simulink model "generic_IVS"  (R2024a)
settings: Solver=FixedStepDiscrete  StartTime=0.0  StopTime=inf  FixedStep=0.001  RelTol=1e-3  EnableMultiTasking=on
undefined symbols (not defined in the file): filtered_route_waypoint_raw, route1_waypoint_x, route1_waypoint_y, route2_waypoint_raw, route2_waypoint_x, route2_waypoint_y, route3_waypoint_x, route3_waypoint_y, route4_waypoint_x, route4_waypoint_y, route5_waypoint_x, route5_waypoint_y
libraries: CarMaker4SL x125, slpidlib x7, simulink x1, robotalgslib x1
(part 3 of 5)

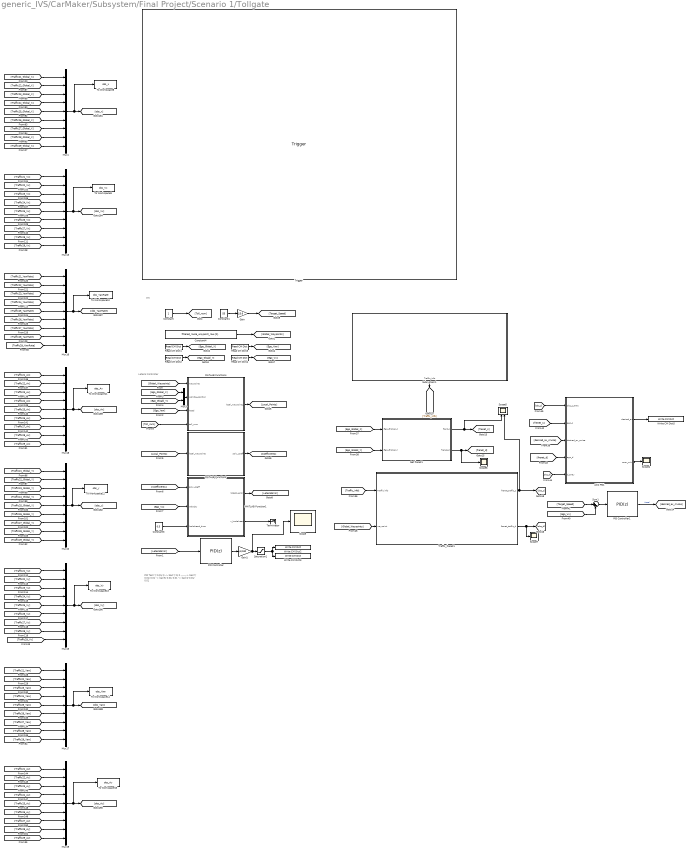
== system generic_IVS/CarMaker/Subsystem/Final Project/Scenario 1/Tollgate ==
  note: Lateral Controller
  note: Init
  note: PID Test
      | 7/ 0.01/ 0 -> bad
      | 7/ 0/ 0 ------> bad
      | 7/ 0.01/ 0.01 -> bad
      | 5/ 0.01/ 0.01 -> bad
      | 3/ 0.01/ 0.01
  Trigger : TriggerPort  TriggerType=function-call  VariantControl=(inherit)  PortDimensions=1
  ACC PD1 : MATLAB Function  TreatAsAtomicUnit=on
  Constant : Constant
  Constant1 : Constant  Value=55
  Constant3 : Constant  Value=0.5
  Constant4 : Constant  Value=filtered_route_waypoint_raw{2}
  Gain : Gain  Gain=1/3.6
  Gain1 : Gain  Gain=pi/180
  Get frenet1 : Subsystem
  MATLAB Function1 : MATLAB Function  TreatAsAtomicUnit=on
  MATLAB Function3 : MATLAB Function  TreatAsAtomicUnit=on
  "MATLAB Function4 " : MATLAB Function  TreatAsAtomicUnit=on
  Mux{1,10,13,15..19} (8 alike) : Mux  Inputs=9
  Mux3 : Mux  Inputs=2
  PID Controller : slpidlib/PID Controller  Controller=PID  Form=Parallel  TimeDomain=Discrete-time  UseExternalTs=off  SampleTime=-1  IntegratorMethod=Forward Euler  FilterMethod=Forward Euler  ControllerParametersSource=internal  P=3  I=0  UseKiTs=off  D=0.01  UseExternalDerivativeSource=off  N=3  UseFilter=on  TunerSelectOption=Transfer Function Based (PID Tuner App)  ZeroCross=off  InitialConditionSource=internal  InitialConditionForIntegrator=0  InitialConditionForFilter=0  DifferentiatorICPrevScaledInput=0  ExternalReset=none  TrackingMode=off  Kt=1  LimitOutput=off  SatLimitsSource=internal  UpperSaturationLimit=inf  LowerSaturationLimit=-inf  LinearizeAsGain=on  AntiWindupMode=none  Kb=1  LimitIntegrator=off  UpperIntegratorSaturationLimit=inf  LowerIntegratorSaturationLimit=-inf  POutMin=[]  POutMax=[]  IOutMin=[]  IOutMax=[]  DOutMin=[]  DOutMax=[]  NOutMin=[]  NOutMax=[]  SumOutMin=[]  SumOutMax=[]  SaturationOutMin=[]  SaturationOutMax=[]  PParamMin=[]  PParamMax=[]  IParamMin=[]  IParamMax=[]  DParamMin=[]  DParamMax=[]  NParamMin=[]  NParamMax=[]  KbParamMin=[]  KbParamMax=[]  KtParamMin=[]  KtParamMax=[]  KbOutMin=[]  KbOutMax=[]  KtOutMin=[]  KtOutMax=[]  IntegratorOutMin=[]  IntegratorOutMax=[]  FilterOutMin=[]  FilterOutMax=[]  SumI1OutMin=[]  SumI1OutMax=[]  SumI2OutMin=[]  SumI2OutMax=[]  SumI3OutMin=[]  SumI3OutMax=[]  SumI4OutMin=[]  SumI4OutMax=[]  SumDOutMin=[]  SumDOutMax=[]  DifferentiatorOutMin=[]  DifferentiatorOutMax=[]  FilterDiffOutCoefMin=[]  FilterDiffOutCoefMax=[]  ReciprocalOutMin=[]  ReciprocalOutMax=[]  SumDenOutMin=[]  SumDenOutMax=[]  SumNumOutMin=[]  SumNumOutMax=[]  DivideOutMin=[]  DivideOutMax=[]  UdiffTsProdOutMin=[]  UdiffTsProdOutMax=[]  NTsProdOutMin=[]  NTsProdOutMax=[]  UintegralTsProdOutMin=[]  UintegralTsProdOutMax=[]  UngainTsProdOutMin=[]  UngainTsProdOutMax=[]  ClampingZeroOutDataTypeStr=Inherit: Inherit via back propagation  ClampingZeroOutMin=[]  ClampingZeroOutMax=[]  FilterDenConstantOutDataTypeStr=Inherit: Inherit via back propagation  FilterDenConstantOutMin=[]  FilterDenConstantOutMax=[]  PCopyOutDataTypeStr=Inherit: Inherit via back propagation  PCopyOutMin=[]  PCopyOutMax=[]  NCopyOutDataTypeStr=Inherit: Inherit via back propagation  NCopyOutMin=[]  NCopyOutMax=[]  IntegratorContinuousStateAttributes=''  IntegratorStateMustResolveToSignalObject=off  IntegratorRTWStateStorageClass=Auto  FilterContinuousStateAttributes=''  FilterStateMustResolveToSignalObject=off  FilterRTWStateStorageClass=Auto  ParallelPVariant=InternalParameters  IdealPVariant=Disabled  IVariant=InternalParameters  DVariant=InternalParameters  IntegratorVariant=Discrete  SatVariant=Disabled  AWVariant=Passthrough  PCopyVariant=Disabled  TRVariant=Disabled  FdbkBlocksVariant=Forward  IdealPFdbkVariant=Disabled  SatFdbkVariant=Disabled  DerivativeFilterVariant=ForwardEulerFilter  NVariant=InternalParameters  NCopyVariant=Disabled  FilterICVariant=InternalICsFilter  IntegratorICVariant=InternalICs  ExternalResetVariant=Disabled  TRSumVariant=Passthrough  SumFdbkVariant=Disabled  SumVariant=Sum_PID  TsampFilterVariant=InternalTs  TsampNgainVariant=Passthrough  TsampIntegralVariant=Disabled_SignalSpec  ExternalSaturationOutDataTypeStr=Inherit: Same as second input  DerivativeSourceVariant=ErrorSignal
  PID Controller1 : slpidlib/PID Controller  Controller=PID  Form=Parallel  TimeDomain=Discrete-time  UseExternalTs=off  SampleTime=-1  IntegratorMethod=Forward Euler  FilterMethod=Forward Euler  ControllerParametersSource=internal  P=1  I=0  UseKiTs=off  D=0  UseExternalDerivativeSource=off  N=20  UseFilter=on  TunerSelectOption=Transfer Function Based (PID Tuner App)  InitialConditionSource=internal  InitialConditionForIntegrator=0  InitialConditionForFilter=0  DifferentiatorICPrevScaledInput=0  ExternalReset=none  TrackingMode=off  Kt=1  LimitOutput=off  SatLimitsSource=internal  UpperSaturationLimit=inf  LowerSaturationLimit=-inf  LinearizeAsGain=on  AntiWindupMode=none  Kb=1  LimitIntegrator=off  UpperIntegratorSaturationLimit=inf  LowerIntegratorSaturationLimit=-inf  POutMin=[]  POutMax=[]  IOutMin=[]  IOutMax=[]  DOutMin=[]  DOutMax=[]  NOutMin=[]  NOutMax=[]  SumOutMin=[]  SumOutMax=[]  SaturationOutMin=[]  SaturationOutMax=[]  PParamMin=[]  PParamMax=[]  IParamMin=[]  IParamMax=[]  DParamMin=[]  DParamMax=[]  NParamMin=[]  NParamMax=[]  KbParamMin=[]  KbParamMax=[]  KtParamMin=[]  KtParamMax=[]  KbOutMin=[]  KbOutMax=[]  KtOutMin=[]  KtOutMax=[]  IntegratorOutMin=[]  IntegratorOutMax=[]  FilterOutMin=[]  FilterOutMax=[]  SumI1OutMin=[]  SumI1OutMax=[]  SumI2OutMin=[]  SumI2OutMax=[]  SumI3OutMin=[]  SumI3OutMax=[]  SumI4OutMin=[]  SumI4OutMax=[]  SumDOutMin=[]  SumDOutMax=[]  DifferentiatorOutMin=[]  DifferentiatorOutMax=[]  FilterDiffOutCoefMin=[]  FilterDiffOutCoefMax=[]  ReciprocalOutMin=[]  ReciprocalOutMax=[]  SumDenOutMin=[]  SumDenOutMax=[]  SumNumOutMin=[]  SumNumOutMax=[]  DivideOutMin=[]  DivideOutMax=[]  UdiffTsProdOutMin=[]  UdiffTsProdOutMax=[]  NTsProdOutMin=[]  NTsProdOutMax=[]  UintegralTsProdOutMin=[]  UintegralTsProdOutMax=[]  UngainTsProdOutMin=[]  UngainTsProdOutMax=[]  ClampingZeroOutDataTypeStr=Inherit: Inherit via back propagation  ClampingZeroOutMin=[]  ClampingZeroOutMax=[]  FilterDenConstantOutDataTypeStr=Inherit: Inherit via back propagation  FilterDenConstantOutMin=[]  FilterDenConstantOutMax=[]  PCopyOutDataTypeStr=Inherit: Inherit via back propagation  PCopyOutMin=[]  PCopyOutMax=[]  NCopyOutDataTypeStr=Inherit: Inherit via back propagation  NCopyOutMin=[]  NCopyOutMax=[]  IntegratorContinuousStateAttributes=''  IntegratorStateMustResolveToSignalObject=off  IntegratorRTWStateStorageClass=Auto  FilterContinuousStateAttributes=''  FilterStateMustResolveToSignalObject=off  FilterRTWStateStorageClass=Auto  ParallelPVariant=InternalParameters  IdealPVariant=Disabled  IVariant=InternalParameters  DVariant=InternalParameters  IntegratorVariant=Discrete  SatVariant=Disabled  AWVariant=Passthrough  PCopyVariant=Disabled  TRVariant=Disabled  FdbkBlocksVariant=Forward  IdealPFdbkVariant=Disabled  SatFdbkVariant=Disabled  DerivativeFilterVariant=ForwardEulerFilter  NVariant=InternalParameters  NCopyVariant=Disabled  FilterICVariant=InternalICsFilter  IntegratorICVariant=InternalICs  ExternalResetVariant=Disabled  TRSumVariant=Passthrough  SumFdbkVariant=Disabled  SumVariant=Sum_PID  TsampFilterVariant=InternalTs  TsampNgainVariant=Passthrough  TsampIntegralVariant=Disabled_SignalSpec  ExternalSaturationOutDataTypeStr=Inherit: Same as second input  DerivativeSourceVariant=ErrorSignal
  Read CM Dict1 : CarMaker4SL/Read CM Dict  xname=Car.Fr1.tx  xsync=off  xstime=Inherited
  Read CM Dict2 : CarMaker4SL/Read CM Dict  xname=Car.Fr1.ty  xsync=off  xstime=Inherited
  Read CM Dict3 : CarMaker4SL/Read CM Dict  xname=Car.Fr1.rz  xsync=off  xstime=Inherited
  Read CM Dict4 : CarMaker4SL/Read CM Dict  xname=Car.v  xsync=off  xstime=Inherited
  Saturation1 : Saturate  UpperLimit=2  LowerLimit=-2
  Scope{,4,6..7} (4 alike) : Scope
  Scope5 : Scope  NumInputPorts=2
  Subsystem1 : Subsystem
  Sum1 : Sum  Inputs=|+-
  Terminator : Terminator
  To Workspace10 : ToWorkspace  VariableName=obs_YawRate  SaveFormat=Timeseries  SampleTime=-1
  To Workspace11 : ToWorkspace  VariableName=obs_Ax  SaveFormat=Timeseries  SampleTime=-1
  To Workspace12 : ToWorkspace  VariableName=obs_y  SaveFormat=Timeseries  SampleTime=-1
  To Workspace13 : ToWorkspace  VariableName=obs_Vy  SaveFormat=Timeseries  SampleTime=-1
  To Workspace14 : ToWorkspace  VariableName=obs_Yaw  SaveFormat=Timeseries  SampleTime=-1
  To Workspace15 : ToWorkspace  VariableName=obs_Ay  SaveFormat=Timeseries  SampleTime=-1
  To Workspace8 : ToWorkspace  VariableName=obs_x  SaveFormat=Timeseries  SampleTime=-1
  To Workspace9 : ToWorkspace  VariableName=obs_Vx  SaveFormat=Timeseries  SampleTime=-1
  Traffic_frenet1 : Subsystem
  Write CM Dict2 : CarMaker4SL/Write CM Dict  xname=Car.CFL.rz_ext  xsync=off
  Write CM Dict3 : CarMaker4SL/Write CM Dict  xname=Car.CFR.rz_ext  xsync=off
  Write CM Dict5 : CarMaker4SL/Write CM Dict  xname=AccelCtrl.DesiredAx  xsync=off
  wires:
  [Ego_Gloabl_Y] -> Mux3/2
  Constant3/1 -> MATLAB Function1/3(lookahead_time)
  Mux3/1 -> "MATLAB Function4 "/2(vehicle_position)
  Gain1/1 -> Scope/1, Saturation1/1
  [Ego_Yaw] -> "MATLAB Function4 "/3(head)
  Read CM Dict2/1 -> [Ego_Gloabl_Y]
  Read CM Dict4/1 -> [Ego_Vx]
  [Global_Waypoints] -> "MATLAB Function4 "/1(waypoints)
  "MATLAB Function4 "/1(local_waypoints_) -> [Local_Points]
  [Coefficients] -> MATLAB Function1/1(poly_coeff)
  MATLAB Function1/2(x_lookahead) -> Terminator/1
  MATLAB Function1/1(lateral_error) -> [LateralError]
  [Local_Points] -> MATLAB Function3/1(local_waypoints)
  PID Controller/1 -> Gain1/1
  [LateralError] -> PID Controller/1
  [Toll_num] -> "MATLAB Function4 "/4(toll_num)
  MATLAB Function3/1(poly_coeff) -> [Coefficients]
  Constant/1 -> [Toll_num]
  Read CM Dict1/1 -> [Ego_Global_X]
  Read CM Dict3/1 -> [Ego_Yaw]
  [Ego_Global_X] -> Mux3/1
  Constant4/1 -> [Global_Waypoints]
  Saturation1/1 -> Write CM Dict2/1, Write CM Dict3/1
  [Ego_Vx] -> MATLAB Function1/2(velocity)
  Constant1/1 -> Gain/1
  Gain/1 -> [Target_Speed]
  [Traffic29_Yaw] -> Mux17/9
  [Traffic28_YawRate] -> Mux16/8
  [Traffic29_YawRate] -> Mux16/9
  [Traffic29_Vy] -> Mux15/9
  [Traffic29_Ay] -> Mux19/9
  [Traffic29_Global_X] -> Mux1/9
  [Traffic29_Vx] -> Mux13/9
  [Traffic29_Ax] -> Mux18/9
  [Traffic29_Global_Y] -> Mux10/9
  Mux13/1 -> To Workspace9/1, [obs_Vx]
  [Traffic21_Vx] -> Mux13/1
  Mux16/1 -> To Workspace10/1, [obs_YawRate]
  [Traffic21_Ax] -> Mux18/1
  [Traffic21_Ay] -> Mux19/1
  [Traffic24_Vx] -> Mux13/4
  [Traffic25_Vy] -> Mux15/5
  [Traffic26_Vx] -> Mux13/6
  [Traffic25_Yaw] -> Mux17/5
  [Traffic25_YawRate] -> Mux16/5
  [Traffic28_Ax] -> Mux18/8
  [Traffic24_Ax] -> Mux18/4
  [Traffic23_Ax] -> Mux18/3
  Mux18/1 -> To Workspace11/1, [obs_Ax]
  [Traffic25_Global_X] -> Mux1/5
  [Traffic26_Global_Y] -> Mux10/6
  Mux10/1 -> To Workspace12/1, [obs_y]
  [Traffic24_Vy] -> Mux15/4
  [Traffic24_Ay] -> Mux19/4
  Mux17/1 -> To Workspace14/1, [obs_Yaw]
  Mux19/1 -> To Workspace15/1, [obs_Ay]
  [Traffic27_YawRate] -> Mux16/7
  [Traffic21_Yaw] -> Mux17/1
  Mux1/1 -> To Workspace8/1, [obs_x]
  [Traffic26_YawRate] -> Mux16/6
  [Traffic23_Global_X] -> Mux1/3
  [Traffic28_Vx] -> Mux13/8
  Mux15/1 -> To Workspace13/1, [obs_Vy]
  [Traffic24_Global_Y] -> Mux10/4
  [Traffic23_Ay] -> Mux19/3
  [Traffic21_Global_Y] -> Mux10/1
  [Traffic27_Ay] -> Mux19/7
  [Traffic22_Ay] -> Mux19/2
  [Traffic27_Vx] -> Mux13/7
  [Traffic22_Yaw] -> Mux17/2
  [Traffic28_Vy] -> Mux15/8
  [Traffic28_Ay] -> Mux19/8
  [Traffic26_Ay] -> Mux19/6
  [Traffic22_Vy] -> Mux15/2
  [Traffic24_Yaw] -> Mux17/4
  [Traffic25_Ax] -> Mux18/5
  [Traffic25_Vx] -> Mux13/5
  [Traffic22_YawRate] -> Mux16/2
  [Traffic27_Ax] -> Mux18/7
  [Traffic27_Vy] -> Mux15/7
  [Traffic26_Yaw] -> Mux17/6
  [Traffic23_Vx] -> Mux13/3
  [Traffic21_Global_X] -> Mux1/1
  [Traffic27_Global_X] -> Mux1/7
  [Traffic27_Yaw] -> Mux17/7
  [Traffic23_Yaw] -> Mux17/3
  [Traffic22_Global_X] -> Mux1/2
  [Traffic28_Yaw] -> Mux17/8
  [Traffic26_Global_X] -> Mux1/6
  [Traffic28_Global_X] -> Mux1/8
  [Traffic22_Vx] -> Mux13/2
  [Traffic26_Vy] -> Mux15/6
  [Traffic24_YawRate] -> Mux16/4
  [Traffic21_YawRate] -> Mux16/1
  [Traffic23_Vy] -> Mux15/3
  [Traffic28_Global_Y] -> Mux10/8
  [Traffic23_Global_Y] -> Mux10/3
  [Traffic26_Ax] -> Mux18/6
  [Traffic27_Global_Y] -> Mux10/7
  [Traffic23_YawRate] -> Mux16/3
  [Traffic21_Vy] -> Mux15/1
  [Traffic22_Global_Y] -> Mux10/2
  [Traffic25_Global_Y] -> Mux10/5
  [Traffic22_Ax] -> Mux18/2
  [Traffic25_Ay] -> Mux19/5
  [Traffic24_Global_X] -> Mux1/4
  Get frenet1/2(frenet_d) -> Scope6/1, [frenet_d]
  [Ego_Gloabl_Y] -> Get frenet1/2(Ego_Global_Y)
  Get frenet1/1(frent_s) -> Scope5/1, [frenet_s]
  [Target_Speed] -> Sum1/1
  [Traffic_info] -> Traffic_frenet1/1(Traffic info)
  Traffic_frenet1/2(frenet_traffic_d) -> Scope7/1, [obs_d]
  ACC PD1/1(desired_ax) -> Write CM Dict5/1
  [frenet_s] -> ACC PD1/2(ego_s)
  [desired_ax_cruise] -> ACC PD1/3(desired_ax_cruise)
  PID Controller1/1 -> [desired_ax_cruise]  "Accel"
  [Global_Waypoints] -> Traffic_frenet1/2(waypoint)
  ACC PD1/2(error_min) -> Scope4/1
  Subsystem1/1(Traffic_Info) -> [Traffic_info]
  [obs_s] -> ACC PD1/1(obs_s_array)
  Traffic_frenet1/1(frenet_traffic_s) -> [obs_s], Scope5/2
  [obs_d] -> ACC PD1/5(d_array)
  Sum1/1 -> PID Controller1/1
  [Ego_Global_X] -> Get frenet1/1(Ego_Global_X)
  [frenet_d] -> ACC PD1/4(ego_d)
  [Ego_Vx] -> Sum1/2

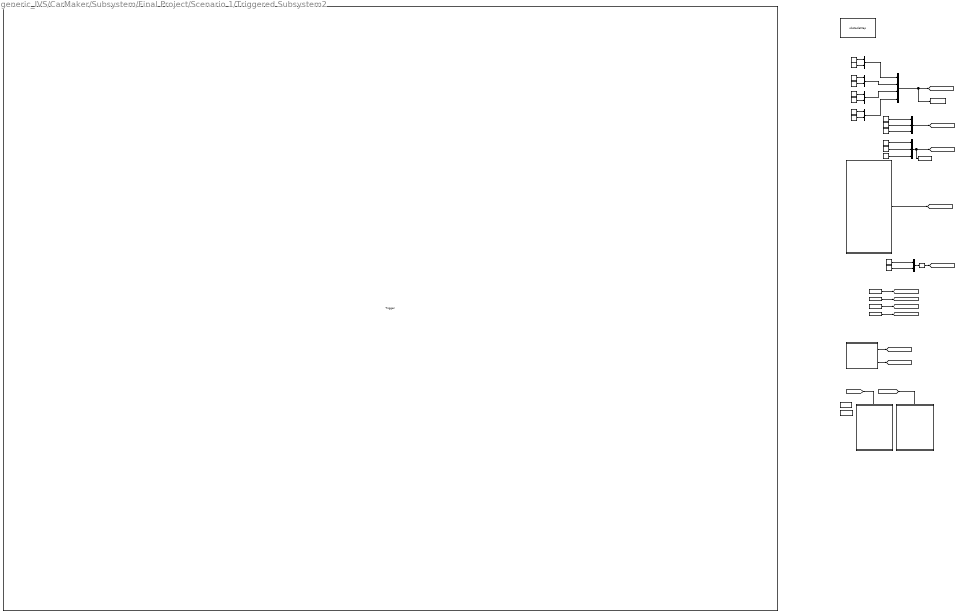
== system generic_IVS/CarMaker/Subsystem/Final Project/Scenario 1/Triggered Subsystem2 ==
  note: Do Not Modify !!
  Trigger : TriggerPort  TriggerType=function-call  VariantControl=(inherit)
      mask Display: image('img.jpg');
  Chart1 : Stateflow chart  TreatAsAtomicUnit=on
      settings: PortSchema="{\"entries\":[{\"content\":{\"sides\":[{\"content\":{},\"type\":\"ConnectorPlacement.EquallySpacedRectSide\",\"uuid\":\"919f2d59-559a-485a-ad64-4ca203985945\"},{\"content\":{\"connectorIds\":[\"Out2\",\"Out1\"],\"side\":\"RIGHT\"},\"type\":\"ConnectorPlacement.EquallySpacedRectSide\",\"uuid\":\"5a15d665-f3e4-404a-9c46-468f267f06f6\"},{\"content\":{\"side\":\"TOP\"},\"type\":\"ConnectorPlacement.EquallySpacedRectSide\",\"uuid\":\"06264e3b-ed7f-4ae7-832b-fa30ed2f7930\"}]},\"type\":\"ConnectorPlacement.EquallySpacedConnector\",\"uuid\":\"55c66715-cf4a-4d9b-b78f-cac3e631d511\"}],\"packageUris\":[\"http://schema.mathworks.com/mf0/Connector/R2020b\"],\"version\":\"1.0\"}"
  Constant1 : Constant  Value=11.5
  Constant10 : Constant  Value=2.48
  Constant2 : Constant  Value=100
  Constant{5..6,24,32,36..37} (6 alike) : Constant  Value=0
  Constant3 : Constant  Value=-100
  Constant30 : Constant  Value=pi/2
  Constant33 : Constant  Value=-20
  Constant34 : Constant  Value=17
  Constant35 : Constant  Value=-6.5
  Constant38 : Constant  Value=-100
  Constant4 : Constant  Value=100
  Data Store Memory : DataStoreMemory  DataStoreName=obstacleMap  WriteAfterWriteMsg=warning  VectorParams1D=off  ShowAdditionalParam=off  Dimensions=[70 3]
  Data Store Memory1 : DataStoreMemory  DataStoreName=orderedPath  WriteAfterWriteMsg=warning  ShowAdditionalParam=off  Dimensions=[300 3]
  Data Store Memory2 : DataStoreMemory  DataStoreName=Finish_p  WriteAfterWriteMsg=warning  ShowAdditionalParam=off  Dimensions=[3 1]
  Data Store Write : DataStoreWrite  DataStoreName=Finish_p  IndexOptions=Index vector (dialog)  Indices=1  OutputSizes=1
  Function-Call Subsystem : Subsystem  TreatAsAtomicUnit=on
  Function-Call Subsystem1 : Subsystem  TreatAsAtomicUnit=on
  Mux10 : Mux  Inputs=3
  Mux{11..12,14..16} (5 alike) : Mux  Inputs=2
  Mux13 : Mux
  Mux3 : Mux  Inputs=3
  Read CM Dict1 : CarMaker4SL/Read CM Dict  xname=Car.Fr1.tx  xsync=off  xstime=Inherited
  Read CM Dict2 : CarMaker4SL/Read CM Dict  xname=Car.Fr1.ty  xsync=off  xstime=Inherited
  Read CM Dict3 : CarMaker4SL/Read CM Dict  xname=Car.Fr1.rz  xsync=off  xstime=Inherited
  Read CM Dict4 : CarMaker4SL/Read CM Dict  xname=Car.v  xsync=off  xstime=Inherited
  Reshape1 : Reshape  OutputDimensionality=Row vector (2-D)  OutputDimensions=[2,2]
  Subsystem : Subsystem
  To Workspace13 : ToWorkspace  VariableName=mapBoundary  SaveFormat=Timeseries  SampleTime=-1
  wires:
  Read CM Dict2/1 -> [Ego_Gloabl_Y]
  Constant2/1 -> Mux15/1
  Constant30/1 -> Mux10/3
  Read CM Dict1/1 -> [Ego_Global_X]
  Constant37/1 -> Mux11/2
  Mux10/1 -> [Finish_Point], Data Store Write/1
  Constant1/1 -> Mux12/2
  Mux11/1 -> Mux13/1
  Constant38/1 -> Mux14/2
  Mux3/1 -> [Start_Point]
  Mux13/1 -> [Map_Boundary], To Workspace13/1
  Constant35/1 -> Mux10/2
  Constant36/1 -> Mux14/1
  [go_Parking] -> Function-Call Subsystem1/Trigger
  Chart1/1(go_Parking()) -> [go_Parking]
  [draw_Map] -> Function-Call Subsystem/Trigger
  Constant10/1 -> Mux12/1
  Constant34/1 -> Mux10/1
  Constant5/1 -> Mux16/2
  Chart1/2(draw_Map()) -> [draw_Map]
  Mux16/1 -> Mux13/2
  Mux12/1 -> Reshape1/1
  Mux14/1 -> Mux13/4
  Constant33/1 -> Mux3/2
  Reshape1/1 -> [Traffic_size]
  Read CM Dict4/1 -> [Ego_Vx]
  Mux15/1 -> Mux13/3
  Read CM Dict3/1 -> [Ego_Yaw]
  Constant3/1 -> Mux15/2
  Constant32/1 -> Mux3/1
  Constant4/1 -> Mux16/1
  Constant24/1 -> Mux3/3
  Subsystem/1(Traffic_Info) -> [Traffic_Info]
  Constant6/1 -> Mux11/1

== system generic_IVS/CarMaker/Subsystem/Final Project/Scenario 1/angle control ==
  Trigger : TriggerPort  TriggerType=function-call  VariantControl=(inherit)
  Add : Sum
  Constant : Constant  Value=4
  Constant1 : Constant  Value=6/3.6
  Constant20 : Constant  Value=route5_waypoint_y.Data
  Constant21 : Constant  Value=route5_waypoint_x.Data
  Gain : Gain  Gain=6
  Gain2 : Gain  Gain=3.6
  Gain3 : Gain  Gain=3.6
  Mux : Mux  Inputs=3
  Mux10 : Mux  Inputs=2
  PID Controller2 : slpidlib/PID Controller  Controller=PID  Form=Parallel  TimeDomain=Discrete-time  UseExternalTs=off  SampleTime=-1  IntegratorMethod=Forward Euler  FilterMethod=Forward Euler  ControllerParametersSource=internal  P=3  I=0  UseKiTs=off  D=0  UseExternalDerivativeSource=off  N=100  UseFilter=on  TunerSelectOption=Transfer Function Based (PID Tuner App)  InitialConditionSource=internal  InitialConditionForIntegrator=0  InitialConditionForFilter=0  DifferentiatorICPrevScaledInput=0  ExternalReset=none  TrackingMode=off  Kt=1  LimitOutput=off  SatLimitsSource=internal  UpperSaturationLimit=inf  LowerSaturationLimit=-inf  LinearizeAsGain=on  AntiWindupMode=none  Kb=1  LimitIntegrator=off  UpperIntegratorSaturationLimit=inf  LowerIntegratorSaturationLimit=-inf  POutMin=[]  POutMax=[]  IOutMin=[]  IOutMax=[]  DOutMin=[]  DOutMax=[]  NOutMin=[]  NOutMax=[]  SumOutMin=[]  SumOutMax=[]  SaturationOutMin=[]  SaturationOutMax=[]  PParamMin=[]  PParamMax=[]  IParamMin=[]  IParamMax=[]  DParamMin=[]  DParamMax=[]  NParamMin=[]  NParamMax=[]  KbParamMin=[]  KbParamMax=[]  KtParamMin=[]  KtParamMax=[]  KbOutMin=[]  KbOutMax=[]  KtOutMin=[]  KtOutMax=[]  IntegratorOutMin=[]  IntegratorOutMax=[]  FilterOutMin=[]  FilterOutMax=[]  SumI1OutMin=[]  SumI1OutMax=[]  SumI2OutMin=[]  SumI2OutMax=[]  SumI3OutMin=[]  SumI3OutMax=[]  SumI4OutMin=[]  SumI4OutMax=[]  SumDOutMin=[]  SumDOutMax=[]  DifferentiatorOutMin=[]  DifferentiatorOutMax=[]  FilterDiffOutCoefMin=[]  FilterDiffOutCoefMax=[]  ReciprocalOutMin=[]  ReciprocalOutMax=[]  SumDenOutMin=[]  SumDenOutMax=[]  SumNumOutMin=[]  SumNumOutMax=[]  DivideOutMin=[]  DivideOutMax=[]  UdiffTsProdOutMin=[]  UdiffTsProdOutMax=[]  NTsProdOutMin=[]  NTsProdOutMax=[]  UintegralTsProdOutMin=[]  UintegralTsProdOutMax=[]  UngainTsProdOutMin=[]  UngainTsProdOutMax=[]  ClampingZeroOutDataTypeStr=Inherit: Inherit via back propagation  ClampingZeroOutMin=[]  ClampingZeroOutMax=[]  FilterDenConstantOutDataTypeStr=Inherit: Inherit via back propagation  FilterDenConstantOutMin=[]  FilterDenConstantOutMax=[]  PCopyOutDataTypeStr=Inherit: Inherit via back propagation  PCopyOutMin=[]  PCopyOutMax=[]  NCopyOutDataTypeStr=Inherit: Inherit via back propagation  NCopyOutMin=[]  NCopyOutMax=[]  IntegratorContinuousStateAttributes=''  IntegratorStateMustResolveToSignalObject=off  IntegratorRTWStateStorageClass=Auto  FilterContinuousStateAttributes=''  FilterStateMustResolveToSignalObject=off  FilterRTWStateStorageClass=Auto  ParallelPVariant=InternalParameters  IdealPVariant=Disabled  IVariant=InternalParameters  DVariant=InternalParameters  IntegratorVariant=Discrete  SatVariant=Disabled  AWVariant=Passthrough  PCopyVariant=Disabled  TRVariant=Disabled  FdbkBlocksVariant=Forward  IdealPFdbkVariant=Disabled  SatFdbkVariant=Disabled  DerivativeFilterVariant=ForwardEulerFilter  NVariant=InternalParameters  NCopyVariant=Disabled  FilterICVariant=InternalICsFilter  IntegratorICVariant=InternalICs  ExternalResetVariant=Disabled  TRSumVariant=Passthrough  SumFdbkVariant=Disabled  SumVariant=Sum_PID  TsampFilterVariant=InternalTs  TsampNgainVariant=Passthrough  TsampIntegralVariant=Disabled_SignalSpec  ExternalSaturationOutDataTypeStr=Inherit: Same as second input  DerivativeSourceVariant=ErrorSignal
  Pure Pursuit : robotalgslib/Pure Pursuit  DesiredLinearVelocityPort=off  DesiredLinearVelocity=5/3.6  MaxAngularVelocity=5.0/3.6  LookaheadDistancePort=off  LookaheadDistance=7  TargetDirPort=off  SimulateUsing=Code generation
  Read CM Dict1 : CarMaker4SL/Read CM Dict  xname=Car.Fr1.tx  xsync=off  xstime=Inherited
  Read CM Dict2 : CarMaker4SL/Read CM Dict  xname=Car.Fr1.ty  xsync=off  xstime=Inherited
  Read CM Dict3 : CarMaker4SL/Read CM Dict  xname=Car.Fr1.rz  xsync=off  xstime=Inherited
  Read CM Dict4 : CarMaker4SL/Read CM Dict  xname=Car.v  xsync=off  xstime=Inherited
  Reshape1 : Reshape  OutputDimensionality=Customize  OutputDimensions=[201, 2]
  Scope1 : Scope
  Scope2 : Scope  NumInputPorts=2
  Sum : Sum  Inputs=|+-
  Terminator : Terminator
  Write CM Dict1 : CarMaker4SL/Write CM Dict  xname=Car.CFL.rz_ext  xsync=off
  Write CM Dict2 : CarMaker4SL/Write CM Dict  xname=Car.CFR.rz_ext  xsync=off
  Write CM Dict3 : CarMaker4SL/Write CM Dict  xname=AccelCtrl.DesiredAx  xsync=off
  wires:
  PID Controller2/1 -> Write CM Dict3/1  "Accel"
  Sum/1 -> PID Controller2/1
  [Ego_Vx] -> Gain3/1, Sum/2
  Gain3/1 -> Scope2/2  "ego"
  [Ego_Yaw] -> Mux/3
  Mux/1 -> Pure Pursuit/1
  [Ego_Global_X] -> Mux/1
  Gain2/1 -> Scope2/1  "target"
  Constant1/1 -> [Target_Velocity]
  [Ego_Gloabl_Y] -> Mux/2
  Read CM Dict4/1 -> [Ego_Vx]
  Read CM Dict1/1 -> [Ego_Global_X]
  Read CM Dict3/1 -> [Ego_Yaw]
  [Target_Velocity] -> Sum/1, Gain2/1
  Pure Pursuit/1 -> Terminator/1
  Read CM Dict2/1 -> [Ego_Gloabl_Y]
  Mux10/1 -> Reshape1/1
  Reshape1/1 -> Pure Pursuit/2
  Pure Pursuit/2 -> Gain/1  "whieel"
  Constant20/1 -> [route5_waypoint_y]
  Constant21/1 -> [route5_waypoint_x]
  [route5_waypoint_x] -> Add/1
  [route5_waypoint_y] -> Mux10/2
  Constant/1 -> Add/2
  Add/1 -> Mux10/1
  Gain/1 -> Scope1/1, Write CM Dict2/1, Write CM Dict1/1

== system generic_IVS/CarMaker/IPG Vehicle/CarAndTrailer/Forces/Suspension Forces/Suspension External Forces Update ==
  Bus Creator21 : BusCreator  Inputs=6
  Bus Creator22 : BusCreator  Inputs=4
  Bus Creator23 : BusCreator  Inputs=4
  From : From  TagVisibility=global
  Ground{32..39} (8 alike) : Ground
  Out1 : Outport
  wires:
  [D] -> Bus Creator21/4
  Ground36/1 -> Bus Creator22/1
  From/1 -> Bus Creator21/1
  [B] -> Bus Creator21/2
  Ground34/1 -> Bus Creator23/3
  Ground32/1 -> Bus Creator23/1
  [C] -> Bus Creator21/3
  Bus Creator23/1 -> Bus Creator21/5
  Ground33/1 -> Bus Creator23/2
  Bus Creator22/1 -> Bus Creator21/6
  Bus Creator21/1 -> Out1/1
  Ground35/1 -> Bus Creator23/4
  Ground39/1 -> Bus Creator22/4
  Ground38/1 -> Bus Creator22/3
  Ground37/1 -> Bus Creator22/2

== system generic_IVS/CarMaker/IPG Vehicle/CarAndTrailer/Forces/Tires/TireFL ==
  note: Insert your tire model here.
  Sync_In : Inport
  Load : Inport  Port=2
  vxtrans : Inport  Port=3
  vytrans : Inport  Port=4
  Rim_rotv : Inport  Port=5
  Rim_turnv : Inport  Port=6
  InclinAngle : Inport  Port=7
  muRoad : Inport  Port=8
  Ground{1..11} (11 alike) : Ground
  Terminator{,1..6,12} (8 alike) : Terminator
  Slp : Outport  VectorParamsAs1DForOutWhenUnconnected=off
  Alpha : Outport  Port=2  VectorParamsAs1DForOutWhenUnconnected=off
  TurnSlp : Outport  Port=3  VectorParamsAs1DForOutWhenUnconnected=off
  rBelt_eff : Outport  Port=4  VectorParamsAs1DForOutWhenUnconnected=off
  vBelt : Outport  Port=5  VectorParamsAs1DForOutWhenUnconnected=off
  LongFrc : Outport  Port=6  VectorParamsAs1DForOutWhenUnconnected=off
  SideFrc : Outport  Port=7  VectorParamsAs1DForOutWhenUnconnected=off
  LoadFrc : Outport  Port=8  VectorParamsAs1DForOutWhenUnconnected=off
  OverturnTrq : Outport  Port=9  VectorParamsAs1DForOutWhenUnconnected=off
  RollResist : Outport  Port=10  VectorParamsAs1DForOutWhenUnconnected=off
  AlignTrq : Outport  Port=11  VectorParamsAs1DForOutWhenUnconnected=off
  wires:
  Ground11/1 -> vBelt/1
  Ground10/1 -> rBelt_eff/1
  Ground9/1 -> TurnSlp/1
  Rim_turnv/1 -> Terminator6/1
  Sync_In/1 -> Terminator12/1
  Ground2/1 -> Alpha/1
  Ground3/1 -> LongFrc/1
  Ground4/1 -> SideFrc/1
  Ground5/1 -> OverturnTrq/1
  vxtrans/1 -> Terminator1/1
  vytrans/1 -> Terminator2/1
  Rim_rotv/1 -> Terminator3/1
  InclinAngle/1 -> Terminator4/1
  muRoad/1 -> Terminator5/1
  Load/1 -> Terminator/1
  Ground1/1 -> Slp/1
  Ground6/1 -> LoadFrc/1
  Ground7/1 -> RollResist/1
  Ground8/1 -> AlignTrq/1

== system generic_IVS/CarMaker/IPG Vehicle/CarAndTrailer/Forces/Tires/TireFR ==
  note: Insert your tire model here.
  Sync_In : Inport
  Load : Inport  Port=2
  vxtrans : Inport  Port=3
  vytrans : Inport  Port=4
  Rim_rotv : Inport  Port=5
  Rim_turnv : Inport  Port=6
  InclinAngle : Inport  Port=7
  muRoad : Inport  Port=8
  Ground{1..11} (11 alike) : Ground
  Terminator{,1..6,12} (8 alike) : Terminator
  Slp : Outport  VectorParamsAs1DForOutWhenUnconnected=off
  Alpha : Outport  Port=2  VectorParamsAs1DForOutWhenUnconnected=off
  TurnSlp : Outport  Port=3  VectorParamsAs1DForOutWhenUnconnected=off
  rBelt_eff : Outport  Port=4  VectorParamsAs1DForOutWhenUnconnected=off
  vBelt : Outport  Port=5  VectorParamsAs1DForOutWhenUnconnected=off
  LongFrc : Outport  Port=6  VectorParamsAs1DForOutWhenUnconnected=off
  SideFrc : Outport  Port=7  VectorParamsAs1DForOutWhenUnconnected=off
  LoadFrc : Outport  Port=8  VectorParamsAs1DForOutWhenUnconnected=off
  OverturnTrq : Outport  Port=9  VectorParamsAs1DForOutWhenUnconnected=off
  RollResist : Outport  Port=10  VectorParamsAs1DForOutWhenUnconnected=off
  AlignTrq : Outport  Port=11  VectorParamsAs1DForOutWhenUnconnected=off
  wires:
  Ground11/1 -> vBelt/1
  Ground10/1 -> rBelt_eff/1
  Ground9/1 -> TurnSlp/1
  Rim_turnv/1 -> Terminator6/1
  Sync_In/1 -> Terminator12/1
  Ground2/1 -> Alpha/1
  Ground3/1 -> LongFrc/1
  Ground4/1 -> SideFrc/1
  Ground5/1 -> OverturnTrq/1
  vxtrans/1 -> Terminator1/1
  vytrans/1 -> Terminator2/1
  Rim_rotv/1 -> Terminator3/1
  InclinAngle/1 -> Terminator4/1
  muRoad/1 -> Terminator5/1
  Load/1 -> Terminator/1
  Ground1/1 -> Slp/1
  Ground6/1 -> LoadFrc/1
  Ground7/1 -> RollResist/1
  Ground8/1 -> AlignTrq/1

== system generic_IVS/CarMaker/IPG Vehicle/CarAndTrailer/Forces/Tires/TireRL ==
  note: Insert your tire model here.
  Sync_In : Inport
  Load : Inport  Port=2
  vxtrans : Inport  Port=3
  vytrans : Inport  Port=4
  Rim_rotv : Inport  Port=5
  Rim_turnv : Inport  Port=6
  InclinAngle : Inport  Port=7
  muRoad : Inport  Port=8
  Ground{1..11} (11 alike) : Ground
  Terminator{,1..6,12} (8 alike) : Terminator
  Slp : Outport  VectorParamsAs1DForOutWhenUnconnected=off
  Alpha : Outport  Port=2  VectorParamsAs1DForOutWhenUnconnected=off
  TurnSlp : Outport  Port=3  VectorParamsAs1DForOutWhenUnconnected=off
  rBelt_eff : Outport  Port=4  VectorParamsAs1DForOutWhenUnconnected=off
  vBelt : Outport  Port=5  VectorParamsAs1DForOutWhenUnconnected=off
  LongFrc : Outport  Port=6  VectorParamsAs1DForOutWhenUnconnected=off
  SideFrc : Outport  Port=7  VectorParamsAs1DForOutWhenUnconnected=off
  LoadFrc : Outport  Port=8  VectorParamsAs1DForOutWhenUnconnected=off
  OverturnTrq : Outport  Port=9  VectorParamsAs1DForOutWhenUnconnected=off
  RollResist : Outport  Port=10  VectorParamsAs1DForOutWhenUnconnected=off
  AlignTrq : Outport  Port=11  VectorParamsAs1DForOutWhenUnconnected=off
  wires:
  Ground11/1 -> vBelt/1
  Ground10/1 -> rBelt_eff/1
  Ground9/1 -> TurnSlp/1
  Rim_turnv/1 -> Terminator6/1
  Sync_In/1 -> Terminator12/1
  Ground2/1 -> Alpha/1
  Ground3/1 -> LongFrc/1
  Ground4/1 -> SideFrc/1
  Ground5/1 -> OverturnTrq/1
  vxtrans/1 -> Terminator1/1
  vytrans/1 -> Terminator2/1
  Rim_rotv/1 -> Terminator3/1
  InclinAngle/1 -> Terminator4/1
  muRoad/1 -> Terminator5/1
  Load/1 -> Terminator/1
  Ground1/1 -> Slp/1
  Ground6/1 -> LoadFrc/1
  Ground7/1 -> RollResist/1
  Ground8/1 -> AlignTrq/1

== system generic_IVS/CarMaker/IPG Vehicle/CarAndTrailer/Forces/Tires/TireRR ==
  note: Insert your tire model here.
  Sync_In : Inport
  Load : Inport  Port=2
  vxtrans : Inport  Port=3
  vytrans : Inport  Port=4
  Rim_rotv : Inport  Port=5
  Rim_turnv : Inport  Port=6
  InclinAngle : Inport  Port=7
  muRoad : Inport  Port=8
  Ground{1..11} (11 alike) : Ground
  Terminator{,1..6,12} (8 alike) : Terminator
  Slp : Outport  VectorParamsAs1DForOutWhenUnconnected=off
  Alpha : Outport  Port=2  VectorParamsAs1DForOutWhenUnconnected=off
  TurnSlp : Outport  Port=3  VectorParamsAs1DForOutWhenUnconnected=off
  rBelt_eff : Outport  Port=4  VectorParamsAs1DForOutWhenUnconnected=off
  vBelt : Outport  Port=5  VectorParamsAs1DForOutWhenUnconnected=off
  LongFrc : Outport  Port=6  VectorParamsAs1DForOutWhenUnconnected=off
  SideFrc : Outport  Port=7  VectorParamsAs1DForOutWhenUnconnected=off
  LoadFrc : Outport  Port=8  VectorParamsAs1DForOutWhenUnconnected=off
  OverturnTrq : Outport  Port=9  VectorParamsAs1DForOutWhenUnconnected=off
  RollResist : Outport  Port=10  VectorParamsAs1DForOutWhenUnconnected=off
  AlignTrq : Outport  Port=11  VectorParamsAs1DForOutWhenUnconnected=off
  wires:
  Ground11/1 -> vBelt/1
  Ground10/1 -> rBelt_eff/1
  Ground9/1 -> TurnSlp/1
  Rim_turnv/1 -> Terminator6/1
  Sync_In/1 -> Terminator12/1
  Ground2/1 -> Alpha/1
  Ground3/1 -> LongFrc/1
  Ground4/1 -> SideFrc/1
  Ground5/1 -> OverturnTrq/1
  vxtrans/1 -> Terminator1/1
  vytrans/1 -> Terminator2/1
  Rim_rotv/1 -> Terminator3/1
  InclinAngle/1 -> Terminator4/1
  muRoad/1 -> Terminator5/1
  Load/1 -> Terminator/1
  Ground1/1 -> Slp/1
  Ground6/1 -> LoadFrc/1
  Ground7/1 -> RollResist/1
  Ground8/1 -> AlignTrq/1

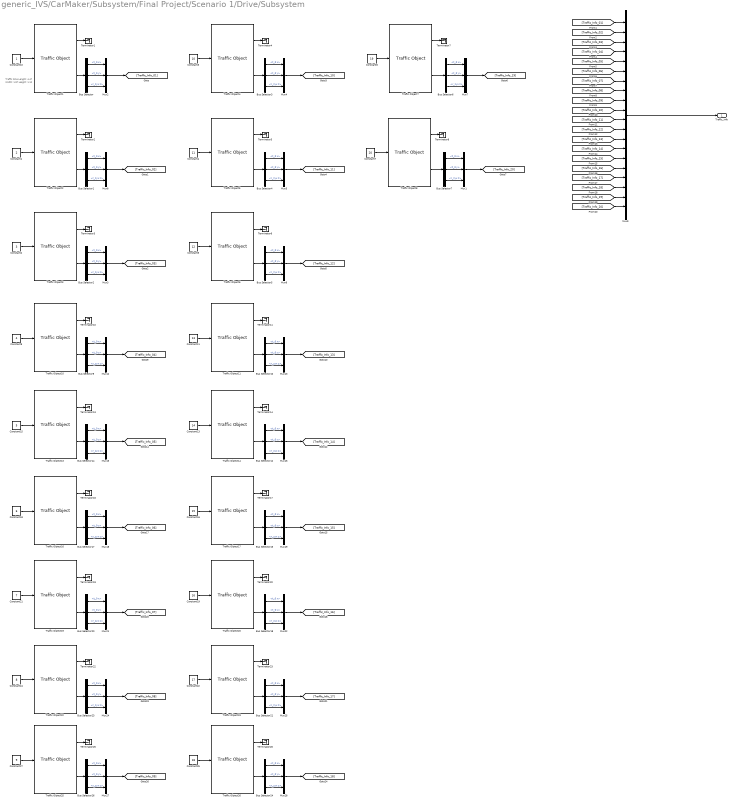
== system generic_IVS/CarMaker/Subsystem/Final Project/Scenario 1/Drive/Subsystem ==
  note: Traffic Size
      | Length: 4.47
      | Width: 1.97
      | Height: 1.12
  Bus Selector{,1..7,9..10,12,14..15,17..18,20..21,23..24,26} (20 alike) : BusSelector  OutputSignals=t_0 x,t_0 y,r_zyx z
  Constant1 : Constant  Value=2
  Constant10 : Constant
  Constant11 : Constant  Value=13
  Constant13 : Constant  Value=14
  Constant15 : Constant  Value=5
  Constant16 : Constant  Value=15
  Constant18 : Constant  Value=6
  Constant19 : Constant  Value=16
  Constant2 : Constant  Value=3
  Constant21 : Constant  Value=7
  Constant22 : Constant  Value=17
  Constant24 : Constant  Value=8
  Constant25 : Constant  Value=18
  Constant27 : Constant  Value=9
  Constant3 : Constant  Value=10
  Constant4 : Constant  Value=11
  Constant5 : Constant  Value=12
  Constant6 : Constant  Value=19
  Constant7 : Constant  Value=20
  Constant9 : Constant  Value=4
  Mux{1..8,12..13,15..16,18..19,21..22,24..25,27..28} (20 alike) : Mux  Inputs=3
  Mux9 : Mux  Inputs=20
  Terminator{1..8,10..11,13..14,16..17,19..20,22..23,25..26} (20 alike) : Terminator
  Traffic Object1 : CarMaker4SL/Traffic Object  xname=T01  ximode=Traffic Id  xstime=Inherited
      settings: SourceProductName=CarMaker4SL
  Traffic Object10 : CarMaker4SL/Traffic Object  xname=T04  ximode=Traffic Id  xstime=Inherited
      settings: SourceProductName=CarMaker4SL
  Traffic Object11 : CarMaker4SL/Traffic Object  xname=T13  ximode=Traffic Id  xstime=Inherited
      settings: SourceProductName=CarMaker4SL
  Traffic Object13 : CarMaker4SL/Traffic Object  xname=T05  ximode=Traffic Id  xstime=Inherited
      settings: SourceProductName=CarMaker4SL
  Traffic Object14 : CarMaker4SL/Traffic Object  xname=T14  ximode=Traffic Id  xstime=Inherited
      settings: SourceProductName=CarMaker4SL
  Traffic Object16 : CarMaker4SL/Traffic Object  xname=T06  ximode=Traffic Id  xstime=Inherited
      settings: SourceProductName=CarMaker4SL
  Traffic Object17 : CarMaker4SL/Traffic Object  xname=T15  ximode=Traffic Id  xstime=Inherited
      settings: SourceProductName=CarMaker4SL
  Traffic Object19 : CarMaker4SL/Traffic Object  xname=T07  ximode=Traffic Id  xstime=Inherited
      settings: SourceProductName=CarMaker4SL
  Traffic Object2 : CarMaker4SL/Traffic Object  xname=T02  ximode=Traffic Id  xstime=Inherited
      settings: SourceProductName=CarMaker4SL
  Traffic Object20 : CarMaker4SL/Traffic Object  xname=T16  ximode=Traffic Id  xstime=Inherited
      settings: SourceProductName=CarMaker4SL
  Traffic Object22 : CarMaker4SL/Traffic Object  xname=T08  ximode=Traffic Id  xstime=Inherited
      settings: SourceProductName=CarMaker4SL
  Traffic Object23 : CarMaker4SL/Traffic Object  xname=T17  ximode=Traffic Id  xstime=Inherited
      settings: SourceProductName=CarMaker4SL
  Traffic Object25 : CarMaker4SL/Traffic Object  xname=T03  ximode=Traffic Id  xstime=Inherited
      settings: SourceProductName=CarMaker4SL
  Traffic Object26 : CarMaker4SL/Traffic Object  xname=T18  ximode=Traffic Id  xstime=Inherited
      settings: SourceProductName=CarMaker4SL
  Traffic Object3 : CarMaker4SL/Traffic Object  xname=T03  ximode=Traffic Id  xstime=Inherited
      settings: SourceProductName=CarMaker4SL
  Traffic Object4 : CarMaker4SL/Traffic Object  xname=T10  ximode=Traffic Id  xstime=Inherited
      settings: SourceProductName=CarMaker4SL
  Traffic Object5 : CarMaker4SL/Traffic Object  xname=T11  ximode=Traffic Id  xstime=Inherited
      settings: SourceProductName=CarMaker4SL
  Traffic Object6 : CarMaker4SL/Traffic Object  xname=T12  ximode=Traffic Id  xstime=Inherited
      settings: SourceProductName=CarMaker4SL
  Traffic Object7 : CarMaker4SL/Traffic Object  xname=T19  ximode=Traffic Id  xstime=Inherited
      settings: SourceProductName=CarMaker4SL
  Traffic Object8 : CarMaker4SL/Traffic Object  xname=T20  ximode=Traffic Id  xstime=Inherited
      settings: SourceProductName=CarMaker4SL
  Traffic_Info : Outport
  wires:
  Constant10/1 -> Traffic Object1/1
  Traffic Object1/1 -> Terminator1/1
  Traffic Object2/1 -> Terminator2/1
  Constant1/1 -> Traffic Object2/1
  Constant2/1 -> Traffic Object3/1
  Traffic Object3/1 -> Terminator3/1
  Traffic Object4/1 -> Terminator4/1
  Constant3/1 -> Traffic Object4/1
  Constant4/1 -> Traffic Object5/1
  Traffic Object5/1 -> Terminator5/1
  Traffic Object6/1 -> Terminator6/1
  Constant5/1 -> Traffic Object6/1
  Constant6/1 -> Traffic Object7/1
  Traffic Object7/1 -> Terminator7/1
  Traffic Object1/2 -> Bus Selector/1
  Bus Selector/1 -> Mux2/1  "<t_0 x>"
  Bus Selector/2 -> Mux2/2  "<t_0 y>"
  Bus Selector/3 -> Mux2/3  "<r_zyx z>"
  Bus Selector1/2 -> Mux8/2  "<t_0 y>"
  Mux8/1 -> [Traffic_Info_02]
  Bus Selector1/1 -> Mux8/1  "<t_0 x>"
  Bus Selector1/3 -> Mux8/3  "<r_zyx z>"
  Traffic Object2/2 -> Bus Selector1/1
  Bus Selector2/2 -> Mux3/2  "<t_0 y>"
  Mux3/1 -> [Traffic_Info_03]
  Bus Selector2/1 -> Mux3/1  "<t_0 x>"
  Bus Selector2/3 -> Mux3/3  "<r_zyx z>"
  Traffic Object3/2 -> Bus Selector2/1
  Bus Selector3/2 -> Mux4/2  "<t_0 y>"
  Mux4/1 -> [Traffic_Info_10]
  Bus Selector3/1 -> Mux4/1  "<t_0 x>"
  Bus Selector3/3 -> Mux4/3  "<r_zyx z>"
  Traffic Object4/2 -> Bus Selector3/1
  Bus Selector4/2 -> Mux5/2  "<t_0 y>"
  Mux5/1 -> [Traffic_Info_11]
  Bus Selector4/1 -> Mux5/1  "<t_0 x>"
  Bus Selector4/3 -> Mux5/3  "<r_zyx z>"
  Traffic Object5/2 -> Bus Selector4/1
  Bus Selector5/2 -> Mux6/2  "<t_0 y>"
  Mux6/1 -> [Traffic_Info_12]
  Bus Selector5/1 -> Mux6/1  "<t_0 x>"
  Bus Selector5/3 -> Mux6/3  "<r_zyx z>"
  Traffic Object6/2 -> Bus Selector5/1
  Bus Selector6/2 -> Mux7/2  "<t_0 y>"
  Mux7/1 -> [Traffic_Info_19]
  Bus Selector6/1 -> Mux7/1  "<t_0 x>"
  Bus Selector6/3 -> Mux7/3  "<r_zyx z>"
  Traffic Object7/2 -> Bus Selector6/1
  Mux2/1 -> [Traffic_Info_01]
  Mux9/1 -> Traffic_Info/1
  Bus Selector7/3 -> Mux1/3  "<r_zyx z>"
  Traffic Object8/2 -> Bus Selector7/1
  Bus Selector7/2 -> Mux1/2  "<t_0 y>"
  Mux1/1 -> [Traffic_Info_20]
  Traffic Object8/1 -> Terminator8/1
  Constant7/1 -> Traffic Object8/1
  Bus Selector7/1 -> Mux1/1  "<t_0 x>"
  Bus Selector10/3 -> Mux13/3  "<r_zyx z>"
  Traffic Object10/2 -> Bus Selector9/1
  Constant11/1 -> Traffic Object11/1
  Bus Selector10/1 -> Mux13/1  "<t_0 x>"
  Traffic Object11/2 -> Bus Selector10/1
  Mux13/1 -> [Traffic_Info_13]
  Bus Selector10/2 -> Mux13/2  "<t_0 y>"
  Mux12/1 -> [Traffic_Info_04]
  Bus Selector9/2 -> Mux12/2  "<t_0 y>"
  Traffic Object11/1 -> Terminator11/1
  Bus Selector9/1 -> Mux12/1  "<t_0 x>"
  Constant9/1 -> Traffic Object10/1
  Traffic Object10/1 -> Terminator10/1
  Bus Selector9/3 -> Mux12/3  "<r_zyx z>"
  Bus Selector14/2 -> Mux15/2  "<t_0 y>"
  Mux15/1 -> [Traffic_Info_05]
  Mux16/1 -> [Traffic_Info_14]
  Traffic Object14/1 -> Terminator14/1
  Bus Selector12/2 -> Mux16/2  "<t_0 y>"
  Traffic Object14/2 -> Bus Selector12/1
  Bus Selector12/1 -> Mux16/1  "<t_0 x>"
  Constant13/1 -> Traffic Object14/1
  Bus Selector12/3 -> Mux16/3  "<r_zyx z>"
  Traffic Object13/2 -> Bus Selector14/1
  Bus Selector14/1 -> Mux15/1  "<t_0 x>"
  Bus Selector14/3 -> Mux15/3  "<r_zyx z>"
  Traffic Object13/1 -> Terminator13/1
  Constant15/1 -> Traffic Object13/1
  Bus Selector17/2 -> Mux18/2  "<t_0 y>"
  Mux18/1 -> [Traffic_Info_06]
  Mux19/1 -> [Traffic_Info_15]
  Traffic Object17/1 -> Terminator17/1
  Bus Selector15/2 -> Mux19/2  "<t_0 y>"
  Traffic Object17/2 -> Bus Selector15/1
  Bus Selector15/1 -> Mux19/1  "<t_0 x>"
  Constant16/1 -> Traffic Object17/1
  Bus Selector15/3 -> Mux19/3  "<r_zyx z>"
  Traffic Object16/2 -> Bus Selector17/1
  Bus Selector17/1 -> Mux18/1  "<t_0 x>"
  Bus Selector17/3 -> Mux18/3  "<r_zyx z>"
  Traffic Object16/1 -> Terminator16/1
  Constant18/1 -> Traffic Object16/1
  Bus Selector20/2 -> Mux21/2  "<t_0 y>"
  Mux21/1 -> [Traffic_Info_07]
  Mux22/1 -> [Traffic_Info_16]
  Traffic Object20/1 -> Terminator20/1
  Bus Selector18/2 -> Mux22/2  "<t_0 y>"
  Traffic Object20/2 -> Bus Selector18/1
  Bus Selector18/1 -> Mux22/1  "<t_0 x>"
  Constant19/1 -> Traffic Object20/1
  Bus Selector18/3 -> Mux22/3  "<r_zyx z>"
  Traffic Object19/2 -> Bus Selector20/1
  Bus Selector20/1 -> Mux21/1  "<t_0 x>"
  Bus Selector20/3 -> Mux21/3  "<r_zyx z>"
  Traffic Object19/1 -> Terminator19/1
  Constant21/1 -> Traffic Object19/1
  Bus Selector23/2 -> Mux24/2  "<t_0 y>"
  Mux24/1 -> [Traffic_Info_08]
  Mux25/1 -> [Traffic_Info_17]
  Traffic Object23/1 -> Terminator23/1
  Bus Selector21/2 -> Mux25/2  "<t_0 y>"
  Traffic Object23/2 -> Bus Selector21/1
  Bus Selector21/1 -> Mux25/1  "<t_0 x>"
  Constant22/1 -> Traffic Object23/1
  Bus Selector21/3 -> Mux25/3  "<r_zyx z>"
  Traffic Object22/2 -> Bus Selector23/1
  Bus Selector23/1 -> Mux24/1  "<t_0 x>"
  Bus Selector23/3 -> Mux24/3  "<r_zyx z>"
  Traffic Object22/1 -> Terminator22/1
  Constant24/1 -> Traffic Object22/1
  Bus Selector26/2 -> Mux27/2  "<t_0 y>"
  Mux27/1 -> [Traffic_Info_09]
  Mux28/1 -> [Traffic_Info_18]
  Traffic Object26/1 -> Terminator26/1
  Bus Selector24/2 -> Mux28/2  "<t_0 y>"
  Traffic Object26/2 -> Bus Selector24/1
  Bus Selector24/1 -> Mux28/1  "<t_0 x>"
  Constant25/1 -> Traffic Object26/1
  Bus Selector24/3 -> Mux28/3  "<r_zyx z>"
  Traffic Object25/2 -> Bus Selector26/1
  Bus Selector26/1 -> Mux27/1  "<t_0 x>"
  Bus Selector26/3 -> Mux27/3  "<r_zyx z>"
  Traffic Object25/1 -> Terminator25/1
  Constant27/1 -> Traffic Object25/1
  [Traffic_Info_01] -> Mux9/1
  [Traffic_Info_02] -> Mux9/2
  [Traffic_Info_03] -> Mux9/3
  [Traffic_Info_04] -> Mux9/4
  [Traffic_Info_05] -> Mux9/5
  [Traffic_Info_06] -> Mux9/6
  [Traffic_Info_07] -> Mux9/7
  [Traffic_Info_08] -> Mux9/8
  [Traffic_Info_09] -> Mux9/9
  [Traffic_Info_10] -> Mux9/10
  [Traffic_Info_11] -> Mux9/11
  [Traffic_Info_12] -> Mux9/12
  [Traffic_Info_13] -> Mux9/13
  [Traffic_Info_14] -> Mux9/14
  [Traffic_Info_15] -> Mux9/15
  [Traffic_Info_16] -> Mux9/16
  [Traffic_Info_17] -> Mux9/17
  [Traffic_Info_18] -> Mux9/18
  [Traffic_Info_19] -> Mux9/19
  [Traffic_Info_20] -> Mux9/20

== system generic_IVS/CarMaker/Subsystem/Final Project/Scenario 1/Tollgate/Get frenet1 ==
  note: Do Not Modify !!
  Ego_Global_X : Inport
  Ego_Global_Y : Inport  Port=2
  Constant1 : Constant  Value=filtered_route_waypoint_raw{2}
  MATLAB Function : MATLAB Function  TreatAsAtomicUnit=on
  MATLAB Function1 : MATLAB Function  TreatAsAtomicUnit=on
  MATLAB Function2 : MATLAB Function  TreatAsAtomicUnit=on
  MATLAB Function3 : MATLAB Function  TreatAsAtomicUnit=on
  MATLAB Function4 : MATLAB Function  TreatAsAtomicUnit=on
  Scope : Scope
  Scope1 : Scope
  Scope3 : Scope
  Terminator : Terminator
  Terminator1 : Terminator
  mapx,mapy2 : Constant  Commented=on  Value=route2_waypoint_raw
  frent_s : Outport
  frenet_d : Outport  Port=2
  wires:
  MATLAB Function1/1(next_wp) -> MATLAB Function2/5(next_wp), Scope3/1
  MATLAB Function3/2(map_y) -> [map_y]
  Constant1/1 -> MATLAB Function3/1(route2_waypoint_raw)
  [Ego_Gloabl_Y] -> MATLAB Function2/2(y)
  [map_y] -> MATLAB Function2/4(mapy)
  MATLAB Function/1(close_wp) -> MATLAB Function1/1(closest_wp)
  [map_x] -> MATLAB Function2/3(mapx)
  [map_y] -> MATLAB Function1/5(mapy)
  [Ego_Global_X] -> MATLAB Function/1(x)
  [Ego_Gloabl_Y] -> MATLAB Function/2(y)
  [map_x] -> MATLAB Function/3(mapx)
  [Ego_Gloabl_Y] -> MATLAB Function1/3(y)
  [Ego_Global_X] -> MATLAB Function2/1(x)
  [Ego_Global_X] -> MATLAB Function1/2(x)
  [map_y] -> MATLAB Function/4(mapy)
  MATLAB Function3/1(map_x) -> [map_x]
  [map_x] -> MATLAB Function1/4(mapx)
  MATLAB Function2/2(frenet_d) -> Scope1/1, frenet_d/1, [frenet_d]
  MATLAB Function2/1(frenet_s) -> [frenet_s]
  MATLAB Function/2(min_len) -> Scope/1
  MATLAB Function4/1(frenet_s_out) -> frent_s/1
  [frenet_s] -> MATLAB Function4/1(frenet_s_in)
  Ego_Global_Y/1 -> [Ego_Gloabl_Y]
  Ego_Global_X/1 -> [Ego_Global_X]
  MATLAB Function2/3(n_x) -> Terminator/1
  MATLAB Function2/4(n_y) -> Terminator1/1

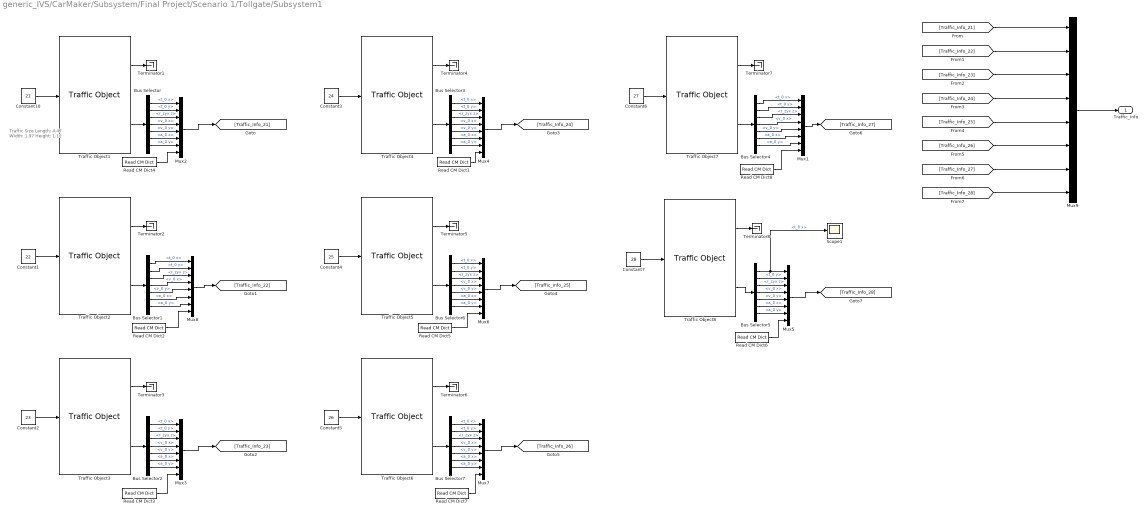
== system generic_IVS/CarMaker/Subsystem/Final Project/Scenario 1/Tollgate/Subsystem1 ==
  note: Traffic Size
      | Length: 4.47
      | Width: 1.97
      | Height: 1.12
  Bus Selector{,1..7} (8 alike) : BusSelector  OutputSignals=t_0 x,t_0 y,r_zyx z,v_0 x,v_0 y,a_0 x,a_0 y
  Constant1 : Constant  Value=22
  Constant10 : Constant  Value=21
  Constant2 : Constant  Value=23
  Constant3 : Constant  Value=24
  Constant4 : Constant  Value=25
  Constant5 : Constant  Value=26
  Constant6 : Constant  Value=27
  Constant7 : Constant  Value=28
  Mux{1..9} (9 alike) : Mux  Inputs=8
  Read CM Dict1 : CarMaker4SL/Read CM Dict  xname=Traffic.T24.rzv  xsync=off  xstime=Inherited
  Read CM Dict2 : CarMaker4SL/Read CM Dict  xname=Traffic.T22.rzv  xsync=off  xstime=Inherited
  Read CM Dict3 : CarMaker4SL/Read CM Dict  xname=Traffic.T23.rzv  xsync=off  xstime=Inherited
  Read CM Dict4 : CarMaker4SL/Read CM Dict  xname=Traffic.T21.rzv  xsync=off  xstime=Inherited
  Read CM Dict5 : CarMaker4SL/Read CM Dict  xname=Traffic.T25.rzv  xsync=off  xstime=Inherited
  Read CM Dict6 : CarMaker4SL/Read CM Dict  xname=Traffic.T28.rzv  xsync=off  xstime=Inherited
  Read CM Dict7 : CarMaker4SL/Read CM Dict  xname=Traffic.T26.rzv  xsync=off  xstime=Inherited
  Read CM Dict8 : CarMaker4SL/Read CM Dict  xname=Traffic.T27.rzv  xsync=off  xstime=Inherited
  Scope1 : Scope
  Terminator{1..8} (8 alike) : Terminator
  Traffic Object1 : CarMaker4SL/Traffic Object  xname=T21  ximode=Traffic Id  xstime=Inherited
      settings: SourceProductName=CarMaker4SL
  Traffic Object2 : CarMaker4SL/Traffic Object  xname=T22  ximode=Traffic Id  xstime=Inherited
      settings: SourceProductName=CarMaker4SL
  Traffic Object3 : CarMaker4SL/Traffic Object  xname=T23  ximode=Traffic Id  xstime=Inherited
      settings: SourceProductName=CarMaker4SL
  Traffic Object4 : CarMaker4SL/Traffic Object  xname=T24  ximode=Traffic Id  xstime=Inherited
      settings: SourceProductName=CarMaker4SL
  Traffic Object5 : CarMaker4SL/Traffic Object  xname=T25  ximode=Traffic Id  xstime=Inherited
      settings: SourceProductName=CarMaker4SL
  Traffic Object6 : CarMaker4SL/Traffic Object  xname=T26  ximode=Traffic Id  xstime=Inherited
      settings: SourceProductName=CarMaker4SL
  Traffic Object7 : CarMaker4SL/Traffic Object  xname=T27  ximode=Traffic Id  xstime=Inherited
      settings: SourceProductName=CarMaker4SL
  Traffic Object8 : CarMaker4SL/Traffic Object  xname=T28  ximode=Traffic Id  xstime=Inherited
      settings: SourceProductName=CarMaker4SL
  Traffic_Info : Outport
  wires:
  Bus Selector7/5 -> Mux7/5  "<v_0 y>"
  Bus Selector7/1 -> Mux7/1  "<t_0 x>"
  Bus Selector7/3 -> Mux7/3  "<r_zyx z>"
  Bus Selector7/7 -> Mux7/7  "<a_0 y>"
  Bus Selector7/2 -> Mux7/2  "<t_0 y>"
  Bus Selector7/4 -> Mux7/4  "<v_0 x>"
  Bus Selector7/6 -> Mux7/6  "<a_0 x>"
  Mux7/1 -> [Traffic_Info_26]
  Traffic Object6/2 -> Bus Selector7/1
  Bus Selector6/5 -> Mux6/5  "<v_0 y>"
  Bus Selector6/1 -> Mux6/1  "<t_0 x>"
  Bus Selector6/3 -> Mux6/3  "<r_zyx z>"
  Bus Selector6/7 -> Mux6/7  "<a_0 y>"
  Bus Selector6/2 -> Mux6/2  "<t_0 y>"
  Bus Selector6/4 -> Mux6/4  "<v_0 x>"
  Bus Selector6/6 -> Mux6/6  "<a_0 x>"
  Mux6/1 -> [Traffic_Info_25]
  Traffic Object5/2 -> Bus Selector6/1
  Bus Selector5/5 -> Mux5/5  "<v_0 y>"
  Bus Selector5/3 -> Mux5/3  "<r_zyx z>"
  Bus Selector5/7 -> Mux5/7  "<a_0 y>"
  Bus Selector5/2 -> Mux5/2  "<t_0 y>"
  Bus Selector5/4 -> Mux5/4  "<v_0 x>"
  Bus Selector5/6 -> Mux5/6  "<a_0 x>"
  Mux5/1 -> [Traffic_Info_28]
  Traffic Object8/2 -> Bus Selector5/1
  Bus Selector4/5 -> Mux1/5  "<v_0 y>"
  Bus Selector4/1 -> Mux1/1  "<t_0 x>"
  Bus Selector4/3 -> Mux1/3  "<r_zyx z>"
  Bus Selector4/7 -> Mux1/7  "<a_0 y>"
  Bus Selector4/2 -> Mux1/2  "<t_0 y>"
  Bus Selector4/4 -> Mux1/4  "<v_0 x>"
  Bus Selector4/6 -> Mux1/6  "<a_0 x>"
  Mux1/1 -> [Traffic_Info_27]
  Traffic Object7/2 -> Bus Selector4/1
  Bus Selector3/5 -> Mux4/5  "<v_0 y>"
  Bus Selector3/1 -> Mux4/1  "<t_0 x>"
  Bus Selector3/3 -> Mux4/3  "<r_zyx z>"
  Bus Selector3/7 -> Mux4/7  "<a_0 y>"
  Bus Selector3/2 -> Mux4/2  "<t_0 y>"
  Bus Selector3/4 -> Mux4/4  "<v_0 x>"
  Bus Selector3/6 -> Mux4/6  "<a_0 x>"
  Mux4/1 -> [Traffic_Info_24]
  Traffic Object4/2 -> Bus Selector3/1
  Mux3/1 -> [Traffic_Info_23]
  Bus Selector2/4 -> Mux3/4  "<v_0 x>"
  Bus Selector2/2 -> Mux3/2  "<t_0 y>"
  Bus Selector2/3 -> Mux3/3  "<r_zyx z>"
  Bus Selector2/5 -> Mux3/5  "<v_0 y>"
  Bus Selector2/6 -> Mux3/6  "<a_0 x>"
  Bus Selector2/7 -> Mux3/7  "<a_0 y>"
  Bus Selector2/1 -> Mux3/1  "<t_0 x>"
  Bus Selector1/7 -> Mux8/7  "<a_0 y>"
  Bus Selector1/5 -> Mux8/5  "<v_0 y>"
  Bus Selector1/3 -> Mux8/3  "<r_zyx z>"
  Bus Selector1/4 -> Mux8/4  "<v_0 x>"
  Bus Selector1/1 -> Mux8/1  "<t_0 x>"
  Bus Selector1/2 -> Mux8/2  "<t_0 y>"
  Bus Selector1/6 -> Mux8/6  "<a_0 x>"
  Mux8/1 -> [Traffic_Info_22]
  Bus Selector/7 -> Mux2/7  "<a_0 y>"
  Bus Selector/6 -> Mux2/6  "<a_0 x>"
  Bus Selector/5 -> Mux2/5  "<v_0 y>"
  Bus Selector/4 -> Mux2/4  "<v_0 x>"
  Bus Selector/3 -> Mux2/3  "<r_zyx z>"
  Bus Selector/2 -> Mux2/2  "<t_0 y>"
  Bus Selector/1 -> Mux2/1  "<t_0 x>"
  [Traffic_Info_28] -> Mux9/8
  Constant7/1 -> Traffic Object8/1
  Traffic Object8/1 -> Terminator8/1
  [Traffic_Info_23] -> Mux9/3
  Mux9/1 -> Traffic_Info/1
  [Traffic_Info_22] -> Mux9/2
  [Traffic_Info_21] -> Mux9/1
  Mux2/1 -> [Traffic_Info_21]
  Traffic Object3/2 -> Bus Selector2/1
  Traffic Object2/2 -> Bus Selector1/1
  Traffic Object1/2 -> Bus Selector/1
  [Traffic_Info_27] -> Mux9/7
  [Traffic_Info_26] -> Mux9/6
  [Traffic_Info_25] -> Mux9/5
  [Traffic_Info_24] -> Mux9/4
  Traffic Object7/1 -> Terminator7/1
  Constant6/1 -> Traffic Object7/1
  Constant5/1 -> Traffic Object6/1
  Traffic Object6/1 -> Terminator6/1
  Traffic Object5/1 -> Terminator5/1
  Constant4/1 -> Traffic Object5/1
  Constant3/1 -> Traffic Object4/1
  Traffic Object4/1 -> Terminator4/1
  Traffic Object3/1 -> Terminator3/1
  Constant2/1 -> Traffic Object3/1
  Constant1/1 -> Traffic Object2/1
  Traffic Object2/1 -> Terminator2/1
  Traffic Object1/1 -> Terminator1/1
  Constant10/1 -> Traffic Object1/1
  Read CM Dict4/1 -> Mux2/8
  Read CM Dict2/1 -> Mux8/8
  Read CM Dict3/1 -> Mux3/8
  Read CM Dict1/1 -> Mux4/8
  Read CM Dict5/1 -> Mux6/8
  Read CM Dict7/1 -> Mux7/8
  Read CM Dict8/1 -> Mux1/8
  Read CM Dict6/1 -> Mux5/8
  Bus Selector5/1 -> Scope1/1, Mux5/1  "<t_0 x>"
